simulink model "sim_topic1"  (R2023b)
settings: Solver=FixedStepAuto  StartTime=0.0  StopTime=T_sim  FixedStep=dt_sim  RelTol=1e-3
undefined symbols (not defined in the file): T
settings Model: Creator=user  LastModifiedBy=user

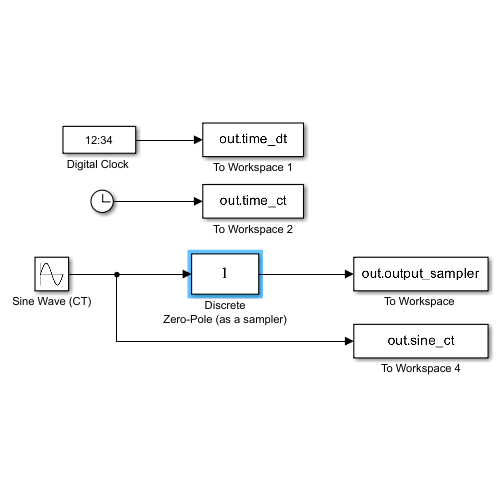
[thumbnail: Simulink's stored preview of the top-level diagram]
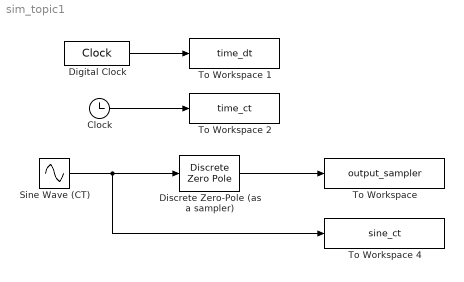
== system sim_topic1 ==
  Clock : Clock
  "Digital Clock " : DigitalClock  SampleTime=T
  Discrete Zero-Pole (as a sampler) : DiscreteZeroPole  Zeros=[]  Poles=[]  Gain=1  SampleTime=T
  Sine Wave (CT) : Sin  Amplitude=3  Frequency=2*pi  SampleTime=0
  "To Workspace " : ToWorkspace  VariableName=output_sampler  SampleTime=T
  To Workspace 1 : ToWorkspace  VariableName=time_dt  SampleTime=T
  To Workspace 2 : ToWorkspace  VariableName=time_ct  SampleTime=-1
  To Workspace 4 : ToWorkspace  VariableName=sine_ct
  wires:
  "Digital Clock "/1 -> To Workspace 1/1
  Clock/1 -> To Workspace 2/1
  Sine Wave (CT)/1 -> To Workspace 4/1, Discrete Zero-Pole (as a sampler)/1
  Discrete Zero-Pole (as a sampler)/1 -> "To Workspace "/1
